simulink model "modelfit"  (R2017b)
settings: Solver=FixedStepAuto  StartTime=0.0  StopTime=10  FixedStep=0.01  RelTol=1e-3
values from neighbouring files (symbols this model uses):
  beta = x(i,j)    [pp_from_simple_model.m]
  g = 9.81    [initialize_simplemodel.m]    (also in initialize_simplemodel_Trial.m; tire_friction_circle.m)
  h = 0.35    [initialize_simplemodel.m]    (also in initialize_simplemodel_Trial.m)
  Izz = 1800    [initialize_simplemodel.m]    (also in initialize_simplemodel_Trial.m = 1400)
  lf = 1.4    [initialize_simplemodel.m]    (also in initialize_simplemodel_Trial.m)
  lr = 1.345    [initialize_simplemodel.m]    (also in initialize_simplemodel_Trial.m)
  m = 1400    [initialize_simplemodel.m]    (also in initialize_simplemodel_Trial.m = 1300; tire_friction_circle.m = 1300)
  r = 0.34    [initialize_simplemodel.m]    (also in initialize_simplemodel_Trial.m)
  tr = 1.684/2    (= 0.842)    [initialize_simplemodel.m]    (also in initialize_simplemodel_Trial.m)
undefined symbols (not defined in the file or in its folder): DiscIntNeverNeededParam, s, t1, t2, t3, t4, v
settings Model: Creator=ashwin.ramanujam  LastModifiedBy=chitr

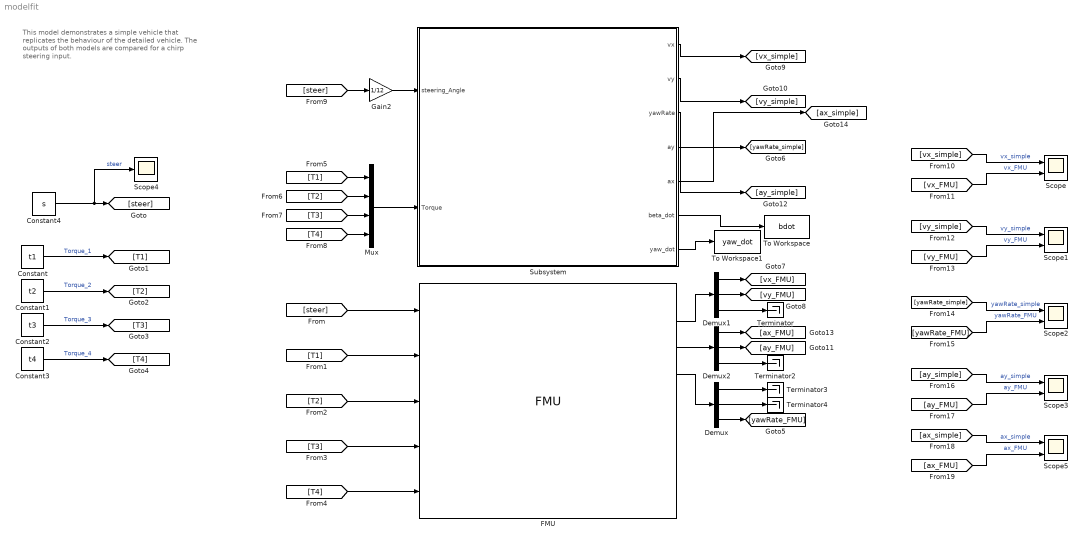
== system modelfit ==
  note: This model demonstrates a simple vehicle that replicates the behaviour of the detailed vehicle. The outputs of both models are compared for a chirp steering input.
  Constant : Constant  Value=t1
  Constant1 : Constant  Value=t2
  Constant2 : Constant  Value=t3
  Constant3 : Constant  Value=t4
  Constant4 : Constant  Value=s
  Demux : Demux  Outputs=3
  Demux1 : Demux  Outputs=3
  Demux2 : Demux  Outputs=3
  FMU : FMU  FMUName=MED2018_VehicleModel.fmu  FMUMode=CoSimulation  FMUSampleTime=-1  mask(MED2018.VehicleModel [Co-Simulation, v2.0]){}
      mask Display:
      | if (exist([Simulink.fileGenControl('get','CacheFolder') '\slprj\_fmu\1f5a25ec6c86b4ef435058314a7136be\MED2018_VehicleModel\model.png'],'file'))
      |     image([Simulink.fileGenControl('get','CacheFolder') '\slprj\_fmu\1f5a25ec6c86b4ef435058314a7136be\MED2018_VehicleModel\model.png']);
      |     text(0.03, 0.97, 'MED2018.VehicleModel', 'horizontalAlignment', 'left', 'verticalAlignment', 'top');
      | else
      |     disp('MED2018.VehicleModel');
      | end
      | port_label('output',1,'Position');
      | port_label('output',2,'Velocity');
      | port_label('output',3,'Acceleration');
      | port_label('output',4,'angularRate');
      | port_label('output',5,'wheelSpeed');
      | port_label('output',6,'wheelTorque_act');
      | port_label('output',7,'offset_Lateral');
      | port_label('output',8,'function_Reward');
      | port_label('output',9,'simulation_State');
      | port_label('input',1,'steering_Angle');
      | port_label('input',2,'wheelTorque_cmd_FL');
      | port_label('input',3,'wheelTorque_cmd_FR');
      | port_label('input',4,'wheelTorque_cmd_RL');
      | port_label('input',5,'wheelTorque_cmd_RR');
  Gain2 : Gain  Gain=1/12
  Mux : Mux
  Scope{,1..3,5} (5 alike) : Scope  NumInputPorts=2
  Scope4 : Scope
  Subsystem : Subsystem
  Terminator{,2..4} (4 alike) : Terminator
  To Workspace : ToWorkspace  VariableName=bdot  SaveFormat=Timeseries  SampleTime=-1
  To Workspace1 : ToWorkspace  VariableName=yaw_dot  SaveFormat=Timeseries  SampleTime=-1
  wires:
  Mux/1 -> Subsystem/2(Torque)
  FMU/4 -> Demux/1
  Demux/3 -> [yawRate_FMU]
  [steer] -> FMU/1
  Constant/1 -> [T1]  "Torque_1"
  Constant1/1 -> [T2]  "Torque_2"
  Constant2/1 -> [T3]  "Torque_3"
  Constant3/1 -> [T4]  "Torque_4"
  [T4] -> FMU/5
  [T1] -> FMU/2
  [T2] -> FMU/3
  [T3] -> FMU/4
  [T1] -> Mux/1
  [T2] -> Mux/2
  [T3] -> Mux/3
  [T4] -> Mux/4
  Subsystem/3(yawRate) -> [yawRate_simple]
  FMU/2 -> Demux1/1
  Demux1/1 -> [vx_FMU]
  Demux1/2 -> [vy_FMU]
  Subsystem/1(vx) -> [vx_simple]
  Subsystem/2(vy) -> [vy_simple]
  [vx_simple] -> Scope/1  "vx_simple"
  [vx_FMU] -> Scope/2  "vx_FMU"
  [vy_FMU] -> Scope1/2  "vy_FMU"
  [vy_simple] -> Scope1/1  "vy_simple"
  [yawRate_FMU] -> Scope2/2  "yawRate_FMU"
  [yawRate_simple] -> Scope2/1  "yawRate_simple"
  Constant4/1 -> Scope4/1, [steer]  "steer"
  [steer] -> Gain2/1
  FMU/3 -> Demux2/1
  Demux2/2 -> [ay_FMU]
  Subsystem/4(ay) -> [ay_simple]
  [ay_FMU] -> Scope3/2  "ay_FMU"
  [ay_simple] -> Scope3/1  "ay_simple"
  Demux1/3 -> Terminator/1
  Demux2/1 -> [ax_FMU]
  Demux2/3 -> Terminator2/1
  Demux/1 -> Terminator3/1
  Demux/2 -> Terminator4/1
  Subsystem/5(ax) -> [ax_simple]
  [ax_simple] -> Scope5/1  "ax_simple"
  [ax_FMU] -> Scope5/2  "ax_FMU"
  Subsystem/6(beta_dot) -> To Workspace/1
  Subsystem/7(yaw_dot) -> To Workspace1/1
  Gain2/1 -> Subsystem/1(steering_Angle)

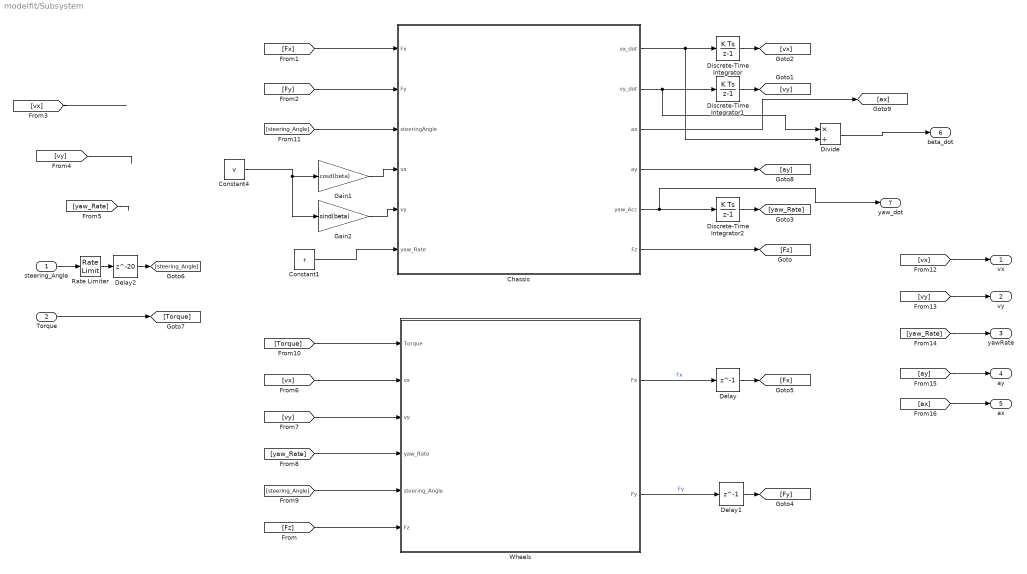
== system modelfit/Subsystem ==
  steering_Angle : Inport
  Torque : Inport  Port=2
  Chassis : MATLAB Function  TreatAsAtomicUnit=on
  Constant1 : Constant  Value=r
  Constant4 : Constant  Value=v
  Delay : Delay  DelayLength=1  InitialCondition=[m*g*lr/(lf+lr)/2;m*g*lr/(lf+lr)/2;m*g*lf/(lf+lr)/2;m*g*lf/(lf+lr)/2]
  Delay1 : Delay  DelayLength=1  InitialCondition=[m*g*lr/(lf+lr)/2;m*g*lr/(lf+lr)/2;m*g*lf/(lf+lr)/2;m*g*lf/(lf+lr)/2]
  Delay2 : Delay  DelayLength=20  InitialCondition=0
  Discrete-Time Integrator : DiscreteIntegrator  InitialCondition=60*5/18  InitialConditionSetting=State (most efficient)  SampleTime=-1  ICPrevOutput=DiscIntNeverNeededParam  ICPrevScaledInput=DiscIntNeverNeededParam
  Discrete-Time Integrator1 : DiscreteIntegrator  InitialConditionSetting=State (most efficient)  SampleTime=-1  ICPrevOutput=DiscIntNeverNeededParam  ICPrevScaledInput=DiscIntNeverNeededParam
  Discrete-Time Integrator2 : DiscreteIntegrator  InitialConditionSetting=State (most efficient)  SampleTime=-1  ICPrevOutput=DiscIntNeverNeededParam  ICPrevScaledInput=DiscIntNeverNeededParam
  Divide : Product  Inputs=*/
  Gain1 : Gain  Gain=cosd(beta)
  Gain2 : Gain  Gain=sind(beta)
  Rate Limiter : RateLimiter  RisingSlewLimit=500*pi/180/12  FallingSlewLimit=-500*pi/180/12  SampleTimeMode=inherited
  Wheels : Subsystem  Priority=0
  vx : Outport
  vy : Outport  Port=2
  yawRate : Outport  Port=3
  ay : Outport  Port=4
  ax : Outport  Port=5
  beta_dot : Outport  Port=6
  yaw_dot : Outport  Port=7
  wires:
  [vx] -> ?
  Discrete-Time Integrator1/1 -> [vy]
  [yaw_Rate] -> ?
  Discrete-Time Integrator/1 -> [vx]
  Discrete-Time Integrator2/1 -> [yaw_Rate]
  [vy] -> ?
  [Fy] -> Chassis/2(Fy)
  [vy] -> Wheels/3(vy)
  [Torque] -> Wheels/1(Torque)
  [yaw_Rate] -> yawRate/1
  [yaw_Rate] -> Wheels/4(yaw_Rate)
  [vx] -> vx/1
  [vx] -> Wheels/2(vx)
  [Fz] -> Wheels/6(Fz)
  [steering_Angle] -> Chassis/3(steeringAngle)
  [steering_Angle] -> Wheels/5(steering_Angle)
  steering_Angle/1 -> Rate Limiter/1
  Torque/1 -> [Torque]
  [vy] -> vy/1
  Chassis/5(yaw_Acc) -> yaw_dot/1, Discrete-Time Integrator2/1
  [Fx] -> Chassis/1(Fx)
  Wheels/1(Fx) -> Delay/1  "Fx"
  Wheels/2(Fy) -> Delay1/1  "Fy"
  Chassis/6(Fz) -> [Fz]
  Rate Limiter/1 -> Delay2/1
  Delay2/1 -> [steering_Angle]
  [ay] -> ay/1
  Delay/1 -> [Fx]
  Delay1/1 -> [Fy]
  Chassis/2(vy_dot) -> Divide/1, Discrete-Time Integrator1/1
  Chassis/4(ay) -> [ay]
  Chassis/3(ax) -> [ax]
  [ax] -> ax/1
  Divide/1 -> beta_dot/1
  Chassis/1(vx_dot) -> Divide/2, Discrete-Time Integrator/1
  Constant4/1 -> Gain2/1, Gain1/1
  Gain1/1 -> Chassis/4(vx)
  Gain2/1 -> Chassis/5(vy)
  Constant1/1 -> Chassis/6(yaw_Rate)

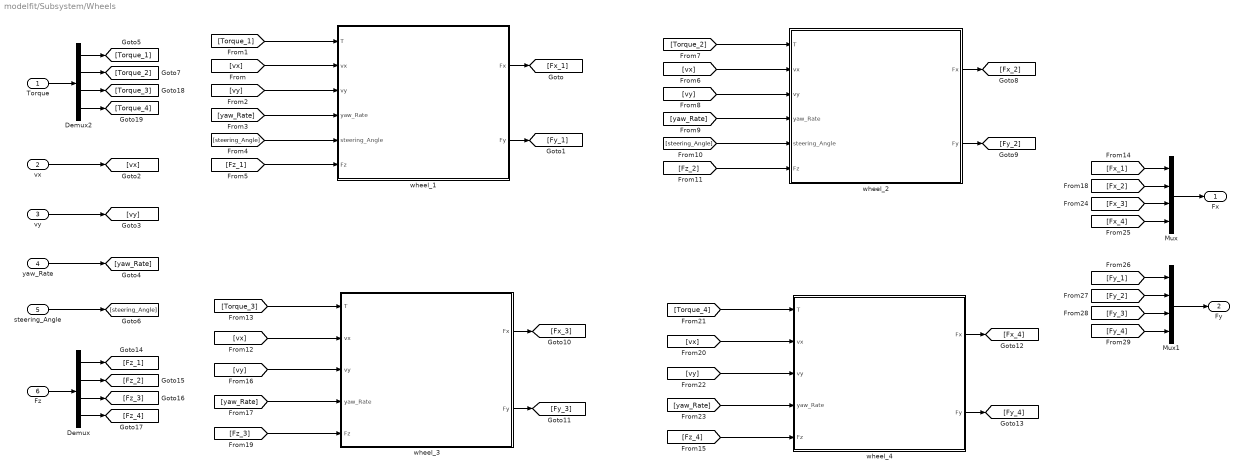
== system modelfit/Subsystem/Wheels ==
  Torque : Inport
  vx : Inport  Port=2
  vy : Inport  Port=3
  yaw_Rate : Inport  Port=4
  steering_Angle : Inport  Port=5
  Fz : Inport  Port=6
  Demux : Demux
  Demux2 : Demux
  Mux : Mux
  Mux1 : Mux
  wheel_1 : Subsystem
  wheel_2 : Subsystem
  wheel_3 : Subsystem
  wheel_4 : Subsystem
  Fx : Outport
  Fy : Outport  Port=2
  wires:
  vx/1 -> [vx]
  vy/1 -> [vy]
  yaw_Rate/1 -> [yaw_Rate]
  [vx] -> wheel_1/2(vx)
  wheel_1/1(Fx) -> [Fx_1]
  wheel_1/2(Fy) -> [Fy_1]
  [steering_Angle] -> wheel_1/5(steering_Angle)
  [yaw_Rate] -> wheel_1/4(yaw_Rate)
  [vy] -> wheel_1/3(vy)
  [Torque_1] -> wheel_1/1(T)
  steering_Angle/1 -> [steering_Angle]
  wheel_2/1(Fx) -> [Fx_2]
  wheel_2/2(Fy) -> [Fy_2]
  [yaw_Rate] -> wheel_2/4(yaw_Rate)
  [vy] -> wheel_2/3(vy)
  [steering_Angle] -> wheel_2/5(steering_Angle)
  [vx] -> wheel_2/2(vx)
  wheel_3/1(Fx) -> [Fx_3]
  [yaw_Rate] -> wheel_3/4(yaw_Rate)
  [vy] -> wheel_4/3(vy)
  [yaw_Rate] -> wheel_4/4(yaw_Rate)
  [vx] -> wheel_4/2(vx)
  wheel_4/2(Fy) -> [Fy_4]
  wheel_3/2(Fy) -> [Fy_3]
  wheel_4/1(Fx) -> [Fx_4]
  [vy] -> wheel_3/3(vy)
  [vx] -> wheel_3/2(vx)
  [Fx_1] -> Mux/1
  [Fx_2] -> Mux/2
  [Fx_3] -> Mux/3
  [Fx_4] -> Mux/4
  [Fy_3] -> Mux1/3
  [Fy_4] -> Mux1/4
  [Fy_2] -> Mux1/2
  [Fy_1] -> Mux1/1
  Demux/1 -> [Fz_1]
  Demux/2 -> [Fz_2]
  Demux/3 -> [Fz_3]
  Demux/4 -> [Fz_4]
  [Fz_1] -> wheel_1/6(Fz)
  [Fz_3] -> wheel_3/5(Fz)
  [Fz_4] -> wheel_4/5(Fz)
  [Fz_2] -> wheel_2/6(Fz)
  Fz/1 -> Demux/1
  [Torque_3] -> wheel_3/1(T)
  [Torque_2] -> wheel_2/1(T)
  [Torque_4] -> wheel_4/1(T)
  Demux2/4 -> [Torque_4]
  Demux2/3 -> [Torque_3]
  Demux2/1 -> [Torque_1]
  Torque/1 -> Demux2/1
  Demux2/2 -> [Torque_2]
  Mux1/1 -> Fy/1
  Mux/1 -> Fx/1

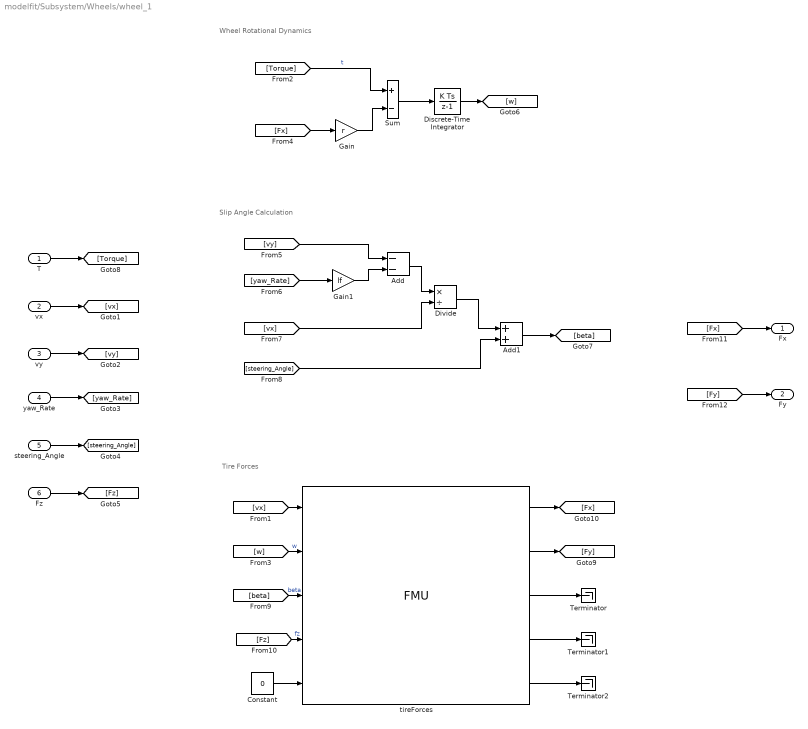
== system modelfit/Subsystem/Wheels/wheel_1 ==
  note: Tire Forces
  note: Wheel Rotational Dynamics
  note: Slip Angle Calculation
  T : Inport
  vx : Inport  Port=2
  vy : Inport  Port=3
  yaw_Rate : Inport  Port=4
  steering_Angle : Inport  Port=5
  Fz : Inport  Port=6
  Add : Sum  Inputs=--
  Add1 : Sum
  Constant : Constant  Value=0
  Discrete-Time Integrator : DiscreteIntegrator  InitialConditionSetting=State (most efficient)  SampleTime=-1  ICPrevOutput=DiscIntNeverNeededParam  ICPrevScaledInput=DiscIntNeverNeededParam
  Divide : Product  Inputs=*/
  Gain : Gain  Gain=r
  Gain1 : Gain  Gain=lf
  Sum : Sum  Inputs=+-
  Terminator : Terminator
  Terminator1 : Terminator
  Terminator2 : Terminator
  tireForces : FMU  FMUName=MED2018_TireModel.fmu  FMUMode=CoSimulation  FMUSampleTime=-1  mask(TyreFMUContainer [Co-Simulation, v2.0]){}
  Fx : Outport
  Fy : Outport  Port=2
  wires:
  Discrete-Time Integrator/1 -> [w]
  tireForces/5 -> Terminator2/1
  tireForces/2 -> [Fy]
  tireForces/4 -> Terminator1/1
  tireForces/3 -> Terminator/1
  Sum/1 -> Discrete-Time Integrator/1
  [Torque] -> Sum/1  "t"
  Gain/1 -> Sum/2
  [Fx] -> Gain/1
  Constant/1 -> tireForces/5
  Gain1/1 -> Add/2
  Add/1 -> Divide/1
  [w] -> tireForces/2  "w"
  vx/1 -> [vx]
  vy/1 -> [vy]
  steering_Angle/1 -> [steering_Angle]
  yaw_Rate/1 -> [yaw_Rate]
  Fz/1 -> [Fz]
  [vx] -> tireForces/1
  [vy] -> Add/1
  [yaw_Rate] -> Gain1/1
  [vx] -> Divide/2
  Divide/1 -> Add1/1
  [steering_Angle] -> Add1/2
  Add1/1 -> [beta]
  [beta] -> tireForces/3  "beta"
  [Fz] -> tireForces/4  "fz"
  T/1 -> [Torque]
  tireForces/1 -> [Fx]
  [Fx] -> Fx/1
  [Fy] -> Fy/1

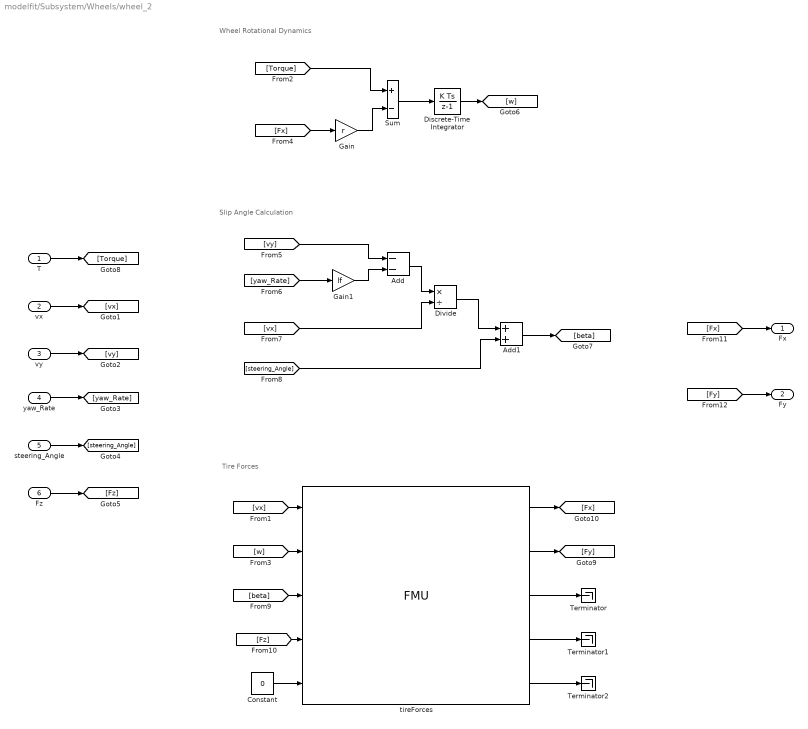
== system modelfit/Subsystem/Wheels/wheel_2 ==
  note: Tire Forces
  note: Wheel Rotational Dynamics
  note: Slip Angle Calculation
  T : Inport
  vx : Inport  Port=2
  vy : Inport  Port=3
  yaw_Rate : Inport  Port=4
  steering_Angle : Inport  Port=5
  Fz : Inport  Port=6
  Add : Sum  Inputs=--
  Add1 : Sum
  Constant : Constant  Value=0
  Discrete-Time Integrator : DiscreteIntegrator  InitialConditionSetting=State (most efficient)  SampleTime=-1  ICPrevOutput=DiscIntNeverNeededParam  ICPrevScaledInput=DiscIntNeverNeededParam
  Divide : Product  Inputs=*/
  Gain : Gain  Gain=r
  Gain1 : Gain  Gain=lf
  Sum : Sum  Inputs=+-
  Terminator : Terminator
  Terminator1 : Terminator
  Terminator2 : Terminator
  tireForces : FMU  FMUName=MED2018_TireModel.fmu  FMUMode=CoSimulation  FMUSampleTime=-1  mask(TyreFMUContainer [Co-Simulation, v2.0]){}
  Fx : Outport
  Fy : Outport  Port=2
  wires:
  Discrete-Time Integrator/1 -> [w]
  tireForces/5 -> Terminator2/1
  tireForces/2 -> [Fy]
  tireForces/4 -> Terminator1/1
  tireForces/3 -> Terminator/1
  Sum/1 -> Discrete-Time Integrator/1
  [Torque] -> Sum/1
  Gain/1 -> Sum/2
  [Fx] -> Gain/1
  Constant/1 -> tireForces/5
  Gain1/1 -> Add/2
  Add/1 -> Divide/1
  [w] -> tireForces/2
  vx/1 -> [vx]
  vy/1 -> [vy]
  steering_Angle/1 -> [steering_Angle]
  yaw_Rate/1 -> [yaw_Rate]
  Fz/1 -> [Fz]
  [vx] -> tireForces/1
  [vy] -> Add/1
  [yaw_Rate] -> Gain1/1
  [vx] -> Divide/2
  Divide/1 -> Add1/1
  [steering_Angle] -> Add1/2
  Add1/1 -> [beta]
  [beta] -> tireForces/3
  [Fz] -> tireForces/4
  T/1 -> [Torque]
  tireForces/1 -> [Fx]
  [Fx] -> Fx/1
  [Fy] -> Fy/1

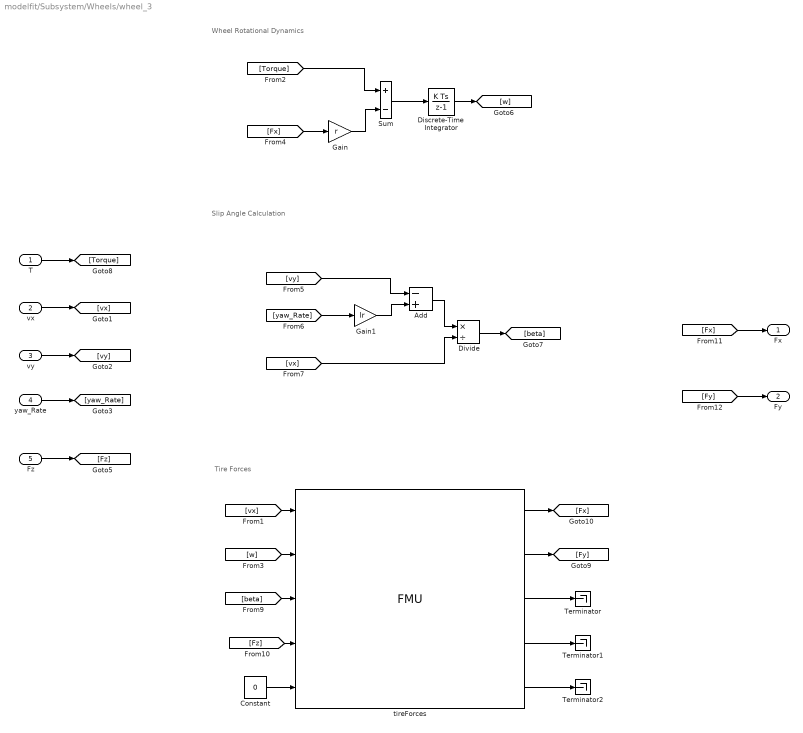
== system modelfit/Subsystem/Wheels/wheel_3 ==
  note: Tire Forces
  note: Wheel Rotational Dynamics
  note: Slip Angle Calculation
  T : Inport
  vx : Inport  Port=2
  vy : Inport  Port=3
  yaw_Rate : Inport  Port=4
  Fz : Inport  Port=5
  Add : Sum  Inputs=-+
  Constant : Constant  Value=0
  Discrete-Time Integrator : DiscreteIntegrator  InitialConditionSetting=State (most efficient)  SampleTime=-1  ICPrevOutput=DiscIntNeverNeededParam  ICPrevScaledInput=DiscIntNeverNeededParam
  Divide : Product  Inputs=*/
  Gain : Gain  Gain=r
  Gain1 : Gain  Gain=lr
  Sum : Sum  Inputs=+-
  Terminator : Terminator
  Terminator1 : Terminator
  Terminator2 : Terminator
  tireForces : FMU  FMUName=MED2018_TireModel.fmu  FMUMode=CoSimulation  FMUSampleTime=-1  mask(TyreFMUContainer [Co-Simulation, v2.0]){}
  Fx : Outport
  Fy : Outport  Port=2
  wires:
  Discrete-Time Integrator/1 -> [w]
  tireForces/5 -> Terminator2/1
  tireForces/2 -> [Fy]
  tireForces/4 -> Terminator1/1
  tireForces/3 -> Terminator/1
  Sum/1 -> Discrete-Time Integrator/1
  [Torque] -> Sum/1
  Gain/1 -> Sum/2
  [Fx] -> Gain/1
  Constant/1 -> tireForces/5
  Gain1/1 -> Add/2
  Add/1 -> Divide/1
  [w] -> tireForces/2
  vx/1 -> [vx]
  vy/1 -> [vy]
  yaw_Rate/1 -> [yaw_Rate]
  Fz/1 -> [Fz]
  [vx] -> tireForces/1
  [vy] -> Add/1
  [yaw_Rate] -> Gain1/1
  [vx] -> Divide/2
  [beta] -> tireForces/3
  [Fz] -> tireForces/4
  T/1 -> [Torque]
  tireForces/1 -> [Fx]
  [Fx] -> Fx/1
  [Fy] -> Fy/1
  Divide/1 -> [beta]

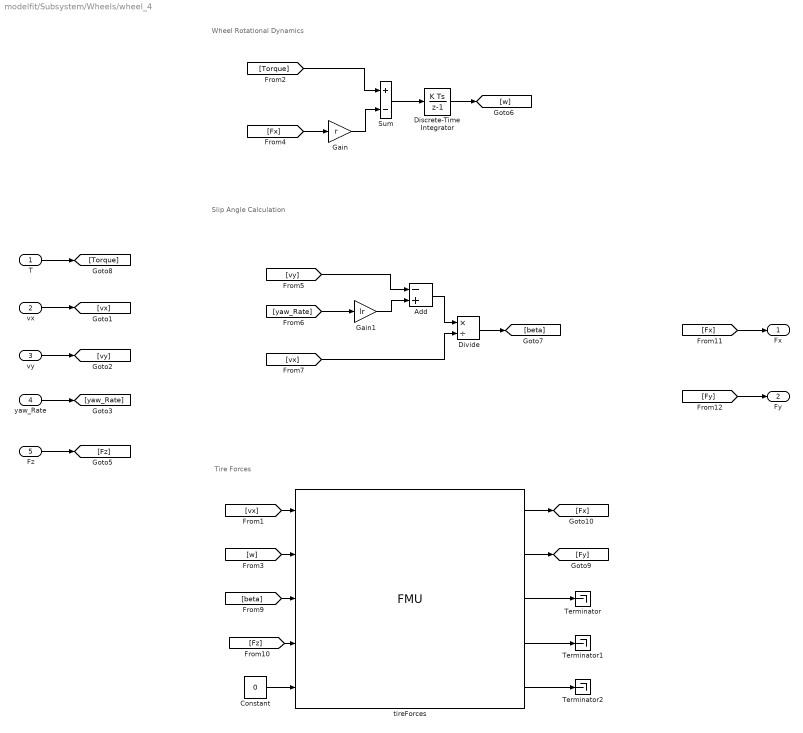
== system modelfit/Subsystem/Wheels/wheel_4 ==
  note: Tire Forces
  note: Wheel Rotational Dynamics
  note: Slip Angle Calculation
  T : Inport
  vx : Inport  Port=2
  vy : Inport  Port=3
  yaw_Rate : Inport  Port=4
  Fz : Inport  Port=5
  Add : Sum  Inputs=-+
  Constant : Constant  Value=0
  Discrete-Time Integrator : DiscreteIntegrator  InitialConditionSetting=State (most efficient)  SampleTime=-1  ICPrevOutput=DiscIntNeverNeededParam  ICPrevScaledInput=DiscIntNeverNeededParam
  Divide : Product  Inputs=*/
  Gain : Gain  Gain=r
  Gain1 : Gain  Gain=lr
  Sum : Sum  Inputs=+-
  Terminator : Terminator
  Terminator1 : Terminator
  Terminator2 : Terminator
  tireForces : FMU  FMUName=MED2018_TireModel.fmu  FMUDebugLogging=on  FMUMode=CoSimulation  FMUSampleTime=-1  mask(TyreFMUContainer [Co-Simulation, v2.0]){}
  Fx : Outport
  Fy : Outport  Port=2
  wires:
  Discrete-Time Integrator/1 -> [w]
  tireForces/5 -> Terminator2/1
  tireForces/2 -> [Fy]
  tireForces/4 -> Terminator1/1
  tireForces/3 -> Terminator/1
  Sum/1 -> Discrete-Time Integrator/1
  [Torque] -> Sum/1
  Gain/1 -> Sum/2
  [Fx] -> Gain/1
  Constant/1 -> tireForces/5
  [w] -> tireForces/2
  vx/1 -> [vx]
  vy/1 -> [vy]
  yaw_Rate/1 -> [yaw_Rate]
  Fz/1 -> [Fz]
  [vx] -> tireForces/1
  [beta] -> tireForces/3
  [Fz] -> tireForces/4
  T/1 -> [Torque]
  tireForces/1 -> [Fx]
  [Fx] -> Fx/1
  [Fy] -> Fy/1
  [vy] -> Add/1
  [vx] -> Divide/2
  [yaw_Rate] -> Gain1/1
  Add/1 -> Divide/1
  Gain1/1 -> Add/2
  Divide/1 -> [beta]

== matlab function modelfit/Subsystem/Chassis ==
  data: vx_dot output; vy_dot output; Fx input; Fy input; steeringAngle input; vx input; vy input; yaw_Rate input; ax output; ay output; yaw_Acc output; Fz output; g parameter; h parameter; Izz parameter; lf parameter; lr parameter; m parameter; tf parameter; tr parameter
function [vx_dot, vy_dot, ax, ay, yaw_Acc, Fz] = vehicleModel(Fx, Fy, steeringAngle, vx, vy, yaw_Rate, g, h, Izz, lf, lr, m, tf, tr)

% Function to simulate vehicle body
% Vehicle Parameters must be loaded from init.m

%Model Equations

fx = (Fx(1)+Fx(2))*cos(steeringAngle) - (Fy(1)+Fy(2))*sin(steeringAngle) + Fx(3) + Fx(4);
fy = (Fx(1)+Fx(2))*sin(steeringAngle) + (Fy(1)+Fy(2))*cos(steeringAngle) + Fy(3) + Fy(4);
Mz =  lf*((Fx(1)+Fx(2))*sin(steeringAngle) + (Fy(1)+Fy(2))*cos(steeringAngle))...
    + tf*((-Fx(1)+Fx(2))*cos(steeringAngle) + (Fy(1)-Fy(2))*sin(steeringAngle))...
    - lr*(Fy(3)+Fy(4)) + tr*(-Fx(3)+Fx(4));

ax = fx/m;
ay = fy/m;

vx_dot      = ax + vy*yaw_Rate;
vy_dot      = ay - vx*yaw_Rate;
yaw_Acc = Mz/Izz;

Fz = zeros(4,1);%[m*g*lr/(lf+lr)/2;m*g*lr/(lf+lr)/2;m*g*lf/(lf+lr)/2;m*g*lf/(lf+lr)/2];
Fz(1) = m * (g*lr/(lf+lr)/2 - ax*h/(lf+lr)/2 - ay*h/tf/2);
Fz(2) = m * (g*lr/(lf+lr)/2 - ax*h/(lf+lr)/2 + ay*h/tf/2);
Fz(3) = m * (g*lf/(lf+lr)/2 + ax*h/(lf+lr)/2 - ay*h/tr/2);
Fz(4) = m * (g*lf/(lf+lr)/2 + ax*h/(lf+lr)/2 + ay*h/tr/2);
